simulink model "untitled1"  (R2023b)
settings: Solver=VariableStepAuto  StartTime=0.0  StopTime=10.0  RelTol=1e-3
undefined symbols (not defined in the file or in its folder): a, b, c, d
settings Model: Creator=chris  LastModifiedBy=chris

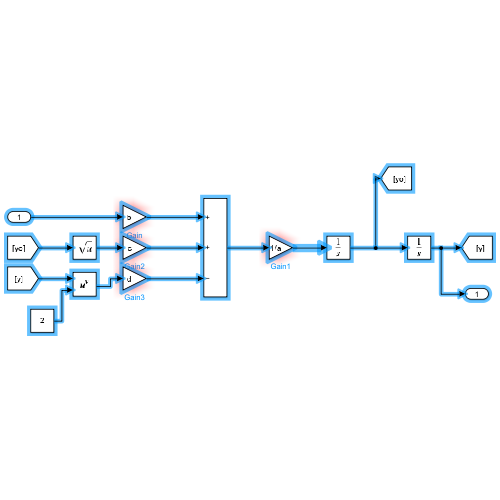
[thumbnail: Simulink's stored preview of the top-level diagram]
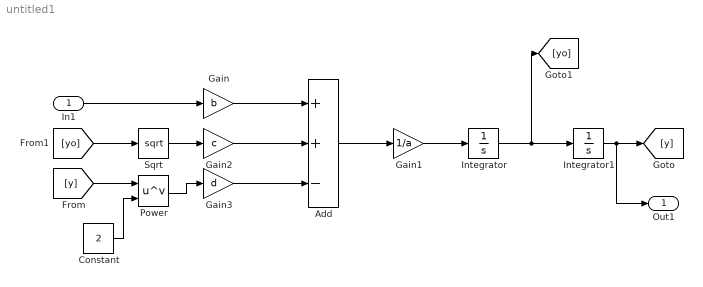
== system untitled1 ==
  In1 : Inport
  Add : Sum  Inputs=++-
  Constant : Constant  Value=2
  Gain : Gain  Gain=b
  Gain1 : Gain  Gain=1/a
  Gain2 : Gain  Gain=c
  Gain3 : Gain  Gain=d
  Integrator : Integrator
  Integrator1 : Integrator
  Power : Math  Operator=pow
  Sqrt : Sqrt
  Out1 : Outport
  wires:
  In1/1 -> Gain/1
  Add/1 -> Gain1/1
  Gain/1 -> Add/1
  Sqrt/1 -> Gain2/1
  Integrator/1 -> [yo], Integrator1/1
  Constant/1 -> Power/2
  [yo] -> Sqrt/1
  Gain2/1 -> Add/2
  Power/1 -> Gain3/1
  Integrator1/1 -> Out1/1, [y]
  [y] -> Power/1
  Gain3/1 -> Add/3
  Gain1/1 -> Integrator/1
